simulink model "controlblackbox"  (R2018b)
settings: Solver=VariableStepAuto  StartTime=0.0  StopTime=10.0  RelTol=1e-3
settings Model: Creator=pizarro  LastModifiedBy=amonp
settings DataIOCC: ReturnWorkspaceOutputs=on

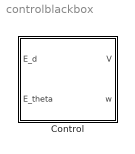
== system controlblackbox ==
  Control : Subsystem

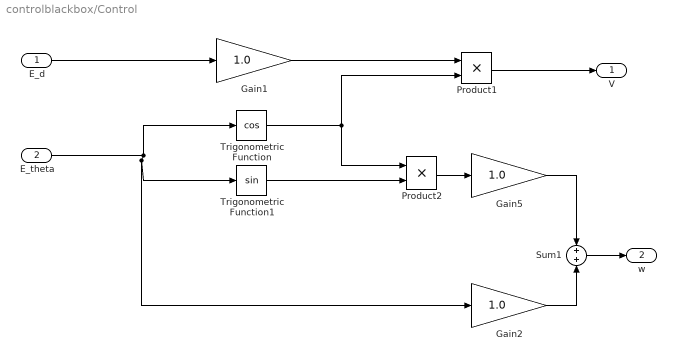
== system controlblackbox/Control ==
  E_d : Inport
  E_theta : Inport  Port=2
  Gain1 : Gain  Gain=1.0
  Gain2 : Gain  Gain=1.0
  Gain5 : Gain  Gain=1.0
  Product1 : Product
  Product2 : Product
  Sum1 : Sum
  Trigonometric Function : Trigonometry  Operator=cos
  Trigonometric Function1 : Trigonometry
  V : Outport  VectorParamsAs1DForOutWhenUnconnected=off
  w : Outport  Port=2  VectorParamsAs1DForOutWhenUnconnected=off
  wires:
  E_theta/1 -> Trigonometric Function/1, Trigonometric Function1/1, Gain2/1
  E_d/1 -> Gain1/1
  Trigonometric Function/1 -> Product1/2, Product2/1
  Product1/1 -> V/1
  Trigonometric Function1/1 -> Product2/2
  Product2/1 -> Gain5/1
  Gain1/1 -> Product1/1
  Gain5/1 -> Sum1/1
  Gain2/1 -> Sum1/2
  Sum1/1 -> w/1
